simulink model "new"  (R2025a)
settings: Solver=VariableStepAuto  StartTime=0.0  StopTime=10.0  RelTol=1e-3
settings Model: Creator=nasim  LastModifiedBy=nasim

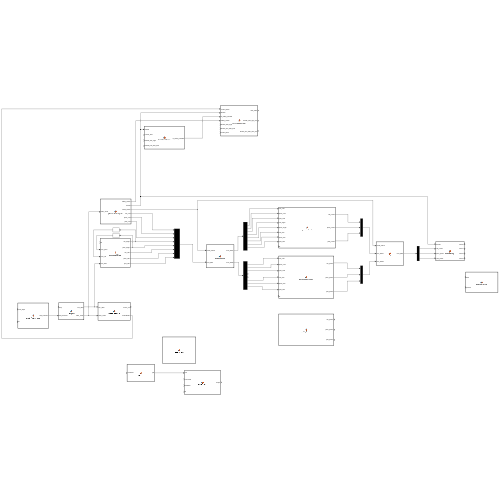
[thumbnail: Simulink's stored preview of the top-level diagram]
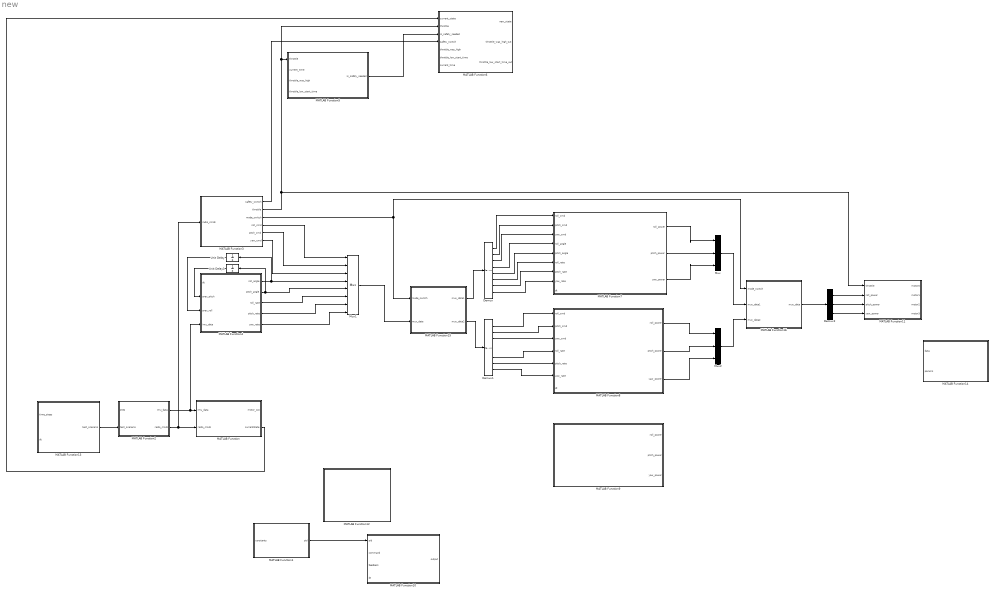
== system new ==
  Demux : Demux  Outputs=8
  Demux1 : Demux  Outputs=8
  Demux2 : Demux  Outputs=3
  MATLAB Function : MATLAB Function  TreatAsAtomicUnit=on
  MATLAB Function1 : MATLAB Function  TreatAsAtomicUnit=on
  MATLAB Function10 : MATLAB Function  TreatAsAtomicUnit=on
  MATLAB Function11 : MATLAB Function  TreatAsAtomicUnit=on
  MATLAB Function12 : MATLAB Function  TreatAsAtomicUnit=on
  MATLAB Function13 : MATLAB Function  TreatAsAtomicUnit=on
  MATLAB Function14 : MATLAB Function  TreatAsAtomicUnit=on
  MATLAB Function15 : MATLAB Function  TreatAsAtomicUnit=on
  MATLAB Function16 : MATLAB Function  TreatAsAtomicUnit=on
  MATLAB Function2 : MATLAB Function  TreatAsAtomicUnit=on
  MATLAB Function3 : MATLAB Function  TreatAsAtomicUnit=on
  MATLAB Function4 : MATLAB Function  TreatAsAtomicUnit=on
  MATLAB Function5 : MATLAB Function  TreatAsAtomicUnit=on
  MATLAB Function6 : MATLAB Function  TreatAsAtomicUnit=on
  MATLAB Function7 : MATLAB Function  TreatAsAtomicUnit=on
  MATLAB Function8 : MATLAB Function  TreatAsAtomicUnit=on
  MATLAB Function9 : MATLAB Function  TreatAsAtomicUnit=on
  Mux : Mux  Inputs=3
  Mux1 : Mux  Inputs=8
  Mux2 : Mux  Inputs=3
  Unit Delay : UnitDelay  SampleTime=-1  HasFrameUpgradeWarning=on
  Unit Delay1 : UnitDelay  SampleTime=-1  HasFrameUpgradeWarning=on
  wires:
  MATLAB Function2/1(imu_data) -> MATLAB Function/1(imu_data), MATLAB Function4/4(imu_data)
  MATLAB Function2/2(radio_cmds) -> MATLAB Function/2(radio_cmds), MATLAB Function3/1(radio_cmds)
  MATLAB Function3/2(throttle) -> MATLAB Function6/2(throttle), MATLAB Function5/1(throttle), MATLAB Function11/1(throttle)
  MATLAB Function/2(currentState) -> MATLAB Function6/1(current_state)
  MATLAB Function5/1(is_safety_needed) -> MATLAB Function6/3(is_safety_needed)
  MATLAB Function3/1(safety_switch) -> MATLAB Function6/4(safety_switch)
  MATLAB Function13/1(test_scenario) -> MATLAB Function2/2(test_scenario)
  MATLAB Function1/1(pid) -> MATLAB Function10/1(pid)
  Mux1/1 -> MATLAB Function15/2(mux_data)
  MATLAB Function3/3(mode_switch) -> MATLAB Function16/1(mode_switch), MATLAB Function15/1(mode_switch)
  MATLAB Function15/1(mux_data1) -> Demux/1
  MATLAB Function15/2(mux_data2) -> Demux1/1
  MATLAB Function7/1(roll_power) -> Mux/1
  MATLAB Function7/2(pitch_power) -> Mux/2
  MATLAB Function7/3(yaw_power) -> Mux/3
  MATLAB Function8/1(roll_power) -> Mux2/1
  MATLAB Function8/2(pitch_power) -> Mux2/2
  MATLAB Function8/3(yaw_power) -> Mux2/3
  MATLAB Function16/1(mux_data) -> Demux2/1
  Demux2/1 -> MATLAB Function11/2(roll_power)
  Demux2/2 -> MATLAB Function11/3(pitch_power)
  Demux2/3 -> MATLAB Function11/4(yaw_power)
  Mux/1 -> MATLAB Function16/2(mux_data1)
  Mux2/1 -> MATLAB Function16/3(mux_data2)
  MATLAB Function3/4(roll_cmd) -> Mux1/1
  MATLAB Function3/5(pitch_cmd) -> Mux1/2
  MATLAB Function3/6(yaw_cmd) -> Mux1/3
  MATLAB Function4/1(roll_angle) -> Mux1/4, Unit Delay/1
  MATLAB Function4/2(pitch_angle) -> Mux1/5, Unit Delay1/1
  MATLAB Function4/3(roll_rate) -> Mux1/6
  MATLAB Function4/4(pitch_rate) -> Mux1/7
  MATLAB Function4/5(yaw_rate) -> Mux1/8
  Demux/2 -> MATLAB Function7/2(pitch_cmd)
  Demux/3 -> MATLAB Function7/3(yaw_cmd)
  Demux/4 -> MATLAB Function7/4(roll_angle)
  Demux/1 -> MATLAB Function7/1(roll_cmd)
  Demux/5 -> MATLAB Function7/5(pitch_angle)
  Demux/6 -> MATLAB Function7/6(roll_rate)
  Demux/7 -> MATLAB Function7/7(pitch_rate)
  Demux/8 -> MATLAB Function7/8(yaw_rate)
  Demux1/1 -> MATLAB Function8/1(roll_cmd)
  Demux1/2 -> MATLAB Function8/2(pitch_cmd)
  Demux1/3 -> MATLAB Function8/3(yaw_cmd)
  Demux1/6 -> MATLAB Function8/4(roll_rate)
  Demux1/7 -> MATLAB Function8/5(pitch_rate)
  Demux1/8 -> MATLAB Function8/6(yaw_rate)
  Unit Delay/1 -> MATLAB Function4/3(prev_roll)
  Unit Delay1/1 -> MATLAB Function4/2(prev_pitch)

== matlab function new/MATLAB Function8 ==
  data: roll_cmd input; pitch_cmd input; yaw_cmd input; roll_rate input; pitch_rate input; yaw_rate input; roll_power output; dt input; pitch_power output; yaw_power output
function [roll_power, pitch_power, yaw_power] = accroModeControl(roll_cmd, pitch_cmd, yaw_cmd,roll_rate, pitch_rate, yaw_rate, dt)
    % Accro mode control - single PID (from Stabilization::Accro)
    persistent rollSpeedPID_Accro pitchSpeedPID_Accro yawPID;
    global params;
    
    if isempty(rollSpeedPID_Accro)
        rollSpeedPID_Accro = initPID(params.accroSpeed);
        pitchSpeedPID_Accro = initPID(params.accroSpeed);
        yawPID = initPID(params.yawSpeed);
    end
    
    % Direct rate control
    roll_power = computePID(rollSpeedPID_Accro, roll_cmd, roll_rate, dt);
    pitch_power = computePID(pitchSpeedPID_Accro, pitch_cmd, pitch_rate, dt);
    yaw_power = computePID(yawPID, yaw_cmd, yaw_rate, dt);
end

== matlab function new/MATLAB Function9 ==
  data: roll_power output; pitch_power output; yaw_power output
function [roll_power, pitch_power, yaw_power] = safetyControl()
    % Safety control - all motors idle (from Stabilization::Idle)
    roll_power = 0;
    pitch_power = 0;
    yaw_power = 0;
    
    % Reset all PID controllers
    resetAllPIDs();
end

== matlab function new/MATLAB Function10 ==
  data: pid input; output output; command input; feedback input; dt input
function output = computePID(pid, command, feedback, dt)
    % Generic PID computation (from ControlLoop::ComputeCorrection)
    error = command - feedback;
    pid.integrator = pid.integrator + error;
    
    output = pid.G * (pid.Kp * error + pid.Kd * (error - pid.prev_error) / dt + pid.Ki * pid.integrator);
    
    pid.prev_error = error;
end

== matlab function new/MATLAB Function11 ==
  data: throttle input; roll_power input; pitch_power input; yaw_power input; motor0 output; motor1 output; motor2 output; motor3 output
function [motor0, motor1, motor2, motor3] = motorMixing(throttle, roll_power, pitch_power, yaw_power)
    % X-configuration motor mixing (from Stabilization::SetMotorsPwrXConfig)
    global params;
    
    % Convert throttle percentage to PWM
    throttle_pwm = params.MOTOR_MIN_POWER + (throttle / 100) * (params.MOTOR_MAX_POWER - params.MOTOR_MIN_POWER);
    
    % X configuration mixing
    motor0 = throttle_pwm - pitch_power * params.mixing + roll_power * params.mixing - yaw_power * params.mixing;
    motor1 = throttle_pwm - pitch_power * params.mixing - roll_power * params.mixing + yaw_power * params.mixing;
    motor2 = throttle_pwm + pitch_power * params.mixing - roll_power * params.mixing - yaw_power * params.mixing;
    motor3 = throttle_pwm + pitch_power * params.mixing + roll_power * params.mixing + yaw_power * params.mixing;
    
    % Apply PWM limits
    motor0 = max(params.MOTOR_MIN_POWER, min(params.MOTOR_MAX_POWER, motor0));
    motor1 = max(params.MOTOR_MIN_POWER, min(params.MOTOR_MAX_POWER, motor1));
    motor2 = max(params.MOTOR_MIN_POWER, min(params.MOTOR_MAX_POWER, motor2));
    motor3 = max(params.MOTOR_MIN_POWER, min(params.MOTOR_MAX_POWER, motor3));
end

== matlab function new/MATLAB Function12 ==
function resetAllPIDs()
    % Reset all PID controllers (from Stabilization::ResetPID)
    persistent rollPosPID pitchPosPID rollSpeedPID_Angle pitchSpeedPID_Angle;
    persistent rollSpeedPID_Accro pitchSpeedPID_Accro yawPID;
    
    if ~isempty(rollPosPID)
        rollPosPID.integrator = 0;
        rollPosPID.prev_error = 0;
    end
    if ~isempty(pitchPosPID)
        pitchPosPID.integrator = 0;
        pitchPosPID.prev_error = 0;
    end
    if ~isempty(rollSpeedPID_Angle)
        rollSpeedPID_Angle.integrator = 0;
        rollSpeedPID_Angle.prev_error = 0;
    end
    if ~isempty(pitchSpeedPID_Angle)
        pitchSpeedPID_Angle.integrator = 0;
        pitchSpeedPID_Angle.prev_error = 0;
    end
    if ~isempty(rollSpeedPID_Accro)
        rollSpeedPID_Accro.integrator = 0;
        rollSpeedPID_Accro.prev_error = 0;
    end
    if ~isempty(pitchSpeedPID_Accro)
        pitchSpeedPID_Accro.integrator = 0;
        pitchSpeedPID_Accro.prev_error = 0;
    end
    if ~isempty(yawPID)
        yawPID.integrator = 0;
        yawPID.prev_error = 0;
    end
end

== matlab function new/MATLAB Function13 ==
  data: time_steps input; test_scenario output; dt input
function test_scenario = createTestScenario(time_steps, dt)
    % Create test scenario with realistic inputs
    time = (0:time_steps-1) * dt;
    
    % Radio commands
    test_scenario.roll_raw = 1500 + 200 * sin(2*pi*0.1*time);     % Slow roll oscillation
    test_scenario.pitch_raw = 1500 + 150 * sin(2*pi*0.15*time);   % Pitch oscillation
    test_scenario.throttle_raw = 1090 + 0 * (time < 5) + 200 * (time >= 5 & time < 15) + 400 * (time >= 15); % Step throttle: 1090->1090->1290->1490
    test_scenario.yaw_raw = 1500 + 100 * sin(2*pi*0.05*time);     % Slow yaw
    test_scenario.mode_raw = 1900 * ones(size(time));             % Angle mode
    test_scenario.safety_raw = 1900 * ones(size(time));           % Armed
    
    % IMU data (simulated)
    test_scenario.acc_x = 0.1 * sin(2*pi*0.1*time);              % Small accelerations
    test_scenario.acc_y = 0.15 * sin(2*pi*0.15*time);
    test_scenario.acc_z = 9.81 + 0.05 * sin(2*pi*0.05*time);     % Gravity + noise
    
    test_scenario.gyro_x = 2 * sin(2*pi*0.1*time);               % Gyro rates
    test_scenario.gyro_y = 1.5 * sin(2*pi*0.15*time);
    test_scenario.gyro_z = 0.5 * sin(2*pi*0.05*time);
end

== matlab function new/MATLAB Function14 ==
  data: data input; params input
function analyzeResults(data, params)
    % Analyze and plot simulation results
    figure('Name', 'CodeDroneDIY Simulation Results', 'Position', [100, 100, 1200, 800]);
    
    % Time vector
    time = data.time;
    
    % Plot 1: Attitude
    subplot(3, 3, 1);
    plot(time, data.roll_angle, 'r-', time, data.pitch_angle, 'b-', 'LineWidth', 2);
    xlabel('Time (s)'); ylabel('Angle (deg)');
    title('Attitude Angles'); legend('Roll', 'Pitch'); grid on;
    
    % Plot 2: Angular Rates
    subplot(3, 3, 2);
    plot(time, data.roll_rate, 'r-', time, data.pitch_rate, 'b-', time, data.yaw_rate, 'g-', 'LineWidth', 2);
    xlabel('Time (s)'); ylabel('Rate (deg/s)');
    title('Angular Rates'); legend('Roll', 'Pitch', 'Yaw'); grid on;
    
    % Plot 3: Commands
    subplot(3, 3, 3);
    plot(time, data.roll_cmd, 'r-', time, data.pitch_cmd, 'b-', 'LineWidth', 2);
    xlabel('Time (s)'); ylabel('Command (deg)');
    title('Control Commands'); legend('Roll Cmd', 'Pitch Cmd'); grid on;
    
    % Plot 4: Throttle
    subplot(3, 3, 4);
    plot(time, data.throttle, 'k-', 'LineWidth', 2);
    xlabel('Time (s)'); ylabel('Throttle (%)');
    title('Throttle'); grid on;
    
    % Plot 5: Motor Outputs
    subplot(3, 3, 5);
    plot(time, data.motor0, 'r-', time, data.motor1, 'g-', time, data.motor2, 'b-', time, data.motor3, 'k-', 'LineWidth', 2);
    xlabel('Time (s)'); ylabel('PWM (us)');
    title('Motor Outputs'); legend('Motor0', 'Motor1', 'Motor2', 'Motor3'); grid on;
    
    % Plot 6: State Machine
    subplot(3, 3, 6);
    plot(time, data.state, 'k-', 'LineWidth', 2);
    xlabel('Time (s)'); ylabel('State');
    title('State Machine'); ylim([0, 6]); grid on;
    
    % Plot 7: Loop Timing
    subplot(3, 3, 7);
    plot(time, data.loop_time * 1000, 'b-', 'LineWidth', 2);
    hold on;
    plot(time, params.LOOP_TIME_TARGET * 1000 * ones(size(time)), 'r--', 'LineWidth', 2);
    xlabel('Time (s)'); ylabel('Loop Time (ms)');
    title('Loop Timing'); legend('Actual', 'Target'); grid on;
    
    % Plot 8: Control Performance
    subplot(3, 3, 8);
    plot(time, data.roll_cmd - data.roll_angle, 'r-', time, data.pitch_cmd - data.pitch_angle, 'b-', 'LineWidth', 2);
    xlabel('Time (s)'); ylabel('Error (deg)');
    title('Control Errors'); legend('Roll Error', 'Pitch Error'); grid on;
    
    % Plot 9: Power Analysis
    subplot(3, 3, 9);
    total_power = data.motor0 + data.motor1 + data.motor2 + data.motor3;
    plot(time, total_power, 'k-', 'LineWidth', 2);
    xlabel('Time (s)'); ylabel('Total Power (us)');
    title('Total Motor Power'); grid on;
    
    % Print performance summary
    fprintf('\n=== PERFORMANCE ANALYSIS ===\n');
    fprintf('RMS Roll Error: %.2f degrees\n', rms(data.roll_cmd - data.roll_angle));
    fprintf('RMS Pitch Error: %.2f degrees\n', rms(data.pitch_cmd - data.pitch_angle));
    fprintf('Mean Loop Time: %.3f ms (Target: %.3f ms)\n', mean(data.loop_time)*1000, params.LOOP_TIME_TARGET*1000);
    fprintf('Loop Time Std: %.3f ms\n', std(data.loop_time)*1000);
    fprintf('Max Loop Time: %.3f ms\n', max(data.loop_time)*1000);
end

== matlab function new/MATLAB Function1 ==
  data: constants input; pid output
function pid = initPID(constants)
    % Initialize PID controller structure
    pid = struct();
    pid.G = constants.G;
    pid.Kp = constants.Kp;
    pid.Kd = constants.Kd;
    pid.Ki = constants.Ki;
    pid.integrator = 0;
    pid.prev_error = 0;
end

== matlab function new/MATLAB Function15 ==
  data: mode_switch input; mux_data1 output; mux_data input; mux_data2 output
function [mux_data1, mux_data2] = modeSelector(mode_switch, mux_data)
% This function routes the input bus 'mux_data' to one of two outputs
% based on the 'mode_switch' signal.

% Ensure the output ports are the same size and type as the input port.
% This is crucial for Simulink to understand the data types.
% coder.varsize('mux_data1', 'mux_data2'); % Optional, but good practice

if mode_switch ~= 0
    % If mode_switch is active (e.g., 1 for Angle Mode),
    % route data to the first output.
    mux_data1 = mux_data;
    
    % The second output receives a zero or empty signal of the same type.
    mux_data2 = 0 * mux_data; % Creates a zero-filled bus of the same structure
else
    % If mode_switch is inactive (0 for Accro Mode),
    % the first output gets the zero signal.
    mux_data1 = 0 * mux_data; 
    
    % Route the data to the second output.
    mux_data2 = mux_data;
end

== matlab function new/MATLAB Function16 ==
  data: mode_switch input; mux_data output; mux_data1 input; mux_data2 input
function mux_data  = modefnc(mode_switch, mux_data1, mux_data2)
if mode_switch ~= 0
    mux_data = mux_data1;
    
else
    mux_data = mux_data2; 
    
end

== matlab function new/MATLAB Function ==
  data: imu_data input; radio_cmds input; motor_out output; currentState output
function [motor_out, currentState] = DroneController(imu_data, radio_cmds)
% This function implements the drone flight controller logic for a single time step.

%#codegen

% Declare persistent variables to hold state between function calls
persistent rollPosPID pitchPosPID rollSpeedPID_Angle pitchSpeedPID_Angle;
persistent rollSpeedPID_Accro pitchSpeedPID_Accro yawPID;
persistent roll_angle_filt pitch_angle_filt;
persistent throttle_was_high throttle_low_start_time;
persistent currentState_internal;

% Load parameters from the base workspace
coder.extrinsic('evalin'); % Allow access to base workspace
params = evalin('base', 'params');

% Initialize all persistent variables on the first run
if isempty(currentState_internal)
    % Initialize PID controllers
    rollPosPID          = initPID(params.anglePos);
    pitchPosPID         = initPID(params.anglePos);
    rollSpeedPID_Angle  = initPID(params.angleSpeed);
    pitchSpeedPID_Angle = initPID(params.angleSpeed);
    rollSpeedPID_Accro  = initPID(params.accroSpeed);
    pitchSpeedPID_Accro = initPID(params.accroSpeed);
    yawPID              = initPID(params.yawSpeed);
    
    % Initialize attitude filter states
    roll_angle_filt     = 0;
    pitch_angle_filt    = 0;
    
    % Initialize safety logic states
    throttle_was_high       = true;
    throttle_low_start_time = 0;
    
    % Initialize state machine
    currentState_internal = params.states.INITIALIZING;
end

% Get simulation time and time step (dt)
current_time = get_param(bdroot, 'SimulationTime');
dt = params.LOOP_TIME_TARGET; % Assumes fixed-step solver

% -------------------- LOGIC FROM YOUR FOR LOOP --------------------

% 1. Process radio inputs
[roll_cmd, pitch_cmd, throttle, yaw_cmd, ~, safety_switch] = processRadioInputs(radio_cmds, params);

% 2. Process IMU data
[roll_angle, pitch_angle, roll_rate, pitch_rate, yaw_rate] = processIMUData(imu_data, dt, roll_angle_filt, pitch_angle_filt, params);

% Update filtered angles for the next time step
roll_angle_filt = roll_angle;
pitch_angle_filt = pitch_angle;

% 3. Check safety conditions
is_safety_needed = checkSafetyState(throttle, current_time, throttle_was_high, throttle_low_start_time);

% 4. Run State Machine
[new_state, throttle_was_high, throttle_low_start_time] = runStateMachine(currentState_internal, throttle, is_safety_needed, safety_switch, throttle_was_high, throttle_low_start_time, current_time, params);
currentState_internal = new_state;

% 5. Run Control Logic based on state
roll_motor_power = 0;
pitch_motor_power = 0;
yaw_motor_power = 0;

switch currentState_internal
    case params.states.ANGLEMODE
        % Angle mode - cascaded PID
        [roll_motor_power, pitch_motor_power, yaw_motor_power] = angleModeControl(...
            roll_cmd, pitch_cmd, yaw_cmd, ...
            roll_angle, pitch_angle, roll_rate, pitch_rate, yaw_rate, dt, ...
            rollPosPID, pitchPosPID, rollSpeedPID_Angle, pitchSpeedPID_Angle, yawPID);
        
    case params.states.ACCRONODE
        % Accro mode - speed PID
        [roll_motor_power, pitch_motor_power, yaw_motor_power] = accroModeControl(...
            roll_cmd, pitch_cmd, yaw_cmd, ...
            roll_rate, pitch_rate, yaw_rate, dt, ...
            rollSpeedPID_Accro, pitchSpeedPID_Accro, yawPID);
        
    case {params.states.SAFETY, params.states.DISARMED, params.states.INITIALIZING}
        % Safety states - reset controllers and output zero power
        [roll_motor_power, pitch_motor_power, yaw_motor_power] = safetyControl();
        % Also reset PID integrators
        rollPosPID.integral = 0; pitchPosPID.integral = 0;
        rollSpeedPID_Angle.integral = 0; pitchSpeedPID_Angle.integral = 0;
        rollSpeedPID_Accro.integral = 0; pitchSpeedPID_Accro.integral = 0;
        yawPID.integral = 0;
end

% 6. X-configuration motor mixing
[m0, m1, m2, m3] = motorMixing(throttle, roll_motor_power, pitch_motor_power, yaw_motor_power, params);

% 7. Assign outputs for the Simulink block
motor_out = [m0; m1; m2; m3];
currentState = currentState_internal;

end


% -------------------- HELPER FUNCTIONS --------------------
% All your other functions (initPID, processRadioInputs, etc.) go here
% as local functions. Make sure they are self-contained.

function pid = initPID(p)
    pid = struct('G', p.G, 'Kp', p.Kp, 'Kd', p.Kd, 'Ki', p.Ki, ...
                 'integral', 0, 'previous_error', 0);
end

function [roll_cmd, pitch_cmd, throttle, yaw_cmd, mode_switch, safety_switch] = processRadioInputs(radio_cmds, params)
    % Dummy function - replace with your actual mapping logic
    throttle = radio_cmds(1); % Assuming throttle is the first channel
    roll_cmd = map_input(radio_cmds(2), params.MAX_ANGLE);
    pitch_cmd = map_input(radio_cmds(3), params.MAX_ANGLE);
    yaw_cmd = map_input(radio_cmds(4), params.MAX_YAW_SPEED);
    mode_switch = radio_cmds(5);
    safety_switch = radio_cmds(6);
end

function out = map_input(value, max_value)
    % Maps a generic input (e.g., 1000-2000) to a physical value
    out = (value - 1500) / 500 * max_value;
end

% ... include all your other helper functions here ...
% e.g., processIMUData, checkSafetyState, runStateMachine, angleModeControl, 
% accroModeControl, safetyControl, motorMixing, etc.

== matlab function new/MATLAB Function2 ==
  data: imu_data output; step input; test_scenario input; radio_cmds output
function [imu_data, radio_cmds] = getInputs(step, test_scenario)
    % Get inputs from test scenario (replace with real sensor data)
    radio_cmds = struct();
    radio_cmds.roll = test_scenario.roll_raw(step);
    radio_cmds.pitch = test_scenario.pitch_raw(step);
    radio_cmds.throttle = test_scenario.throttle_raw(step);
    radio_cmds.yaw = test_scenario.yaw_raw(step);
    radio_cmds.mode = test_scenario.mode_raw(step);
    radio_cmds.safety = test_scenario.safety_raw(step);
    
    imu_data = struct();
    imu_data.acc_x = test_scenario.acc_x(step);
    imu_data.acc_y = test_scenario.acc_y(step);
    imu_data.acc_z = test_scenario.acc_z(step);
    imu_data.gyro_x = test_scenario.gyro_x(step);
    imu_data.gyro_y = test_scenario.gyro_y(step);
    imu_data.gyro_z = test_scenario.gyro_z(step);
end

== matlab function new/MATLAB Function3 ==
  data: safety_switch output; throttle output; mode_switch output; radio_cmds input; roll_cmd output; pitch_cmd output; yaw_cmd output
function [safety_switch, throttle,mode_switch,  roll_cmd, pitch_cmd, yaw_cmd] = processRadioInputs(radio_cmds)
    % Process radio inputs (from RadioReception.cpp)
    global params;
    
    % Scale inputs to match your C++ code
    roll_cmd = (radio_cmds.roll - 1500) * params.MAX_ANGLE / 400;      % ±45 degrees
    pitch_cmd = (radio_cmds.pitch - 1500) * params.MAX_ANGLE / 400;    % ±45 degrees
    throttle = (radio_cmds.throttle - 1090) * 100 / 810; % 0-100%
    yaw_cmd = (radio_cmds.yaw - 1500) * params.MAX_YAW_SPEED / 400;       % ±135 deg/s
    
    % Mode selection
    if radio_cmds.mode > 1700
        mode_switch = 1; % Angle mode
    elseif radio_cmds.mode < 1300
        mode_switch = 0; % Accro mode
    else
        mode_switch = 0; % Default to Accro
    end
    
    % Safety switch
    safety_switch = (radio_cmds.safety > 1500);
    
    % Apply limits
    roll_cmd = max(-params.MAX_ANGLE, min(params.MAX_ANGLE, roll_cmd));
    pitch_cmd = max(-params.MAX_ANGLE, min(params.MAX_ANGLE, pitch_cmd));
    yaw_cmd = max(-params.MAX_YAW_SPEED, min(params.MAX_YAW_SPEED, yaw_cmd));
    throttle = max(0, min(100, throttle));
end

== matlab function new/MATLAB Function4 ==
  data: dt input; prev_pitch input; prev_roll input; imu_data input; roll_angle output; pitch_angle output; roll_rate output; pitch_rate output; yaw_rate output
function [roll_angle, pitch_angle, roll_rate, pitch_rate, yaw_rate] = processIMUData(dt, prev_pitch, prev_roll, imu_data)
    % Process IMU data with complementary filter (from Stabilization.cpp)
    global params;
    
    % Convert gyro to degrees/second
    roll_rate = imu_data.gyro_x;
    pitch_rate = imu_data.gyro_y;
    yaw_rate = imu_data.gyro_z;
    
    % Normalize accelerometer
    acc_mag = sqrt(imu_data.acc_x^2 + imu_data.acc_y^2 + imu_data.acc_z^2);
    acc_x_norm = imu_data.acc_x / acc_mag;
    acc_y_norm = imu_data.acc_y / acc_mag;
    acc_z_norm = imu_data.acc_z / acc_mag;
    
    % Calculate angles from accelerometer
    roll_angle_acc = atan2(acc_y_norm, acc_z_norm) * 180/pi;
    pitch_angle_acc = atan2(-acc_x_norm, acc_z_norm) * 180/pi;
    
    % Complementary filter (from Stabilization::ApplyComplementaryFilter)
    roll_angle = params.HighPassFilterCoeff * (prev_roll + roll_rate * dt) + (1 - params.HighPassFilterCoeff) * roll_angle_acc;
    pitch_angle = params.HighPassFilterCoeff * (prev_pitch + pitch_rate * dt) + (1 - params.HighPassFilterCoeff) * pitch_angle_acc;
end

== matlab function new/MATLAB Function5 ==
  data: throttle input; is_safety_needed output; current_time input; throttle_was_high input; throttle_low_start_time input
function is_safety_needed = checkSafetyState(throttle, current_time, throttle_was_high, throttle_low_start_time)
    % Safety state logic (from StateMachine::IsSafetyStateNeeded)
    global params;
    
    if throttle_was_high && throttle < params.MOTOR_IDLE_THRESHOLD
        is_safety_needed = false;
    elseif ~throttle_was_high && (current_time - throttle_low_start_time > params.SAFETY_TIMEOUT)
        is_safety_needed = true;
    else
        is_safety_needed = false;
    end
end

== matlab function new/MATLAB Function6 ==
  data: current_state input; new_state output; throttle input; is_safety_needed input; safety_switch input; throttle_was_high input; throttle_low_start_time input; current_time input; throttle_was_high_out output; throttle_low_start_time_out output
function [new_state, throttle_was_high_out, throttle_low_start_time_out] = runStateMachine(current_state, throttle, is_safety_needed, safety_switch, throttle_was_high, throttle_low_start_time, current_time)
    % State machine logic (from StateMachine.cpp and state implementations)
    global params;
    
    new_state = current_state;
    throttle_was_high_out = throttle_was_high;
    throttle_low_start_time_out = throttle_low_start_time;
    
    switch current_state
        case params.states.INITIALIZING
            % Transition to Disarmed when IMU is calibrated (from Initializing.cpp)
            % In the C++ code, this transitions to Disarmed, then to AngleMode when throttle high
            new_state = params.states.DISARMED;
            
        case params.states.ANGLEMODE
            if is_safety_needed
                new_state = params.states.SAFETY;
            end
            
        case params.states.ACCRONODE
            if is_safety_needed
                new_state = params.states.SAFETY;
            end
            
        case params.states.SAFETY
            % Automatic transition to disarmed after 1 second
            new_state = params.states.DISARMED;
            
        case params.states.DISARMED
            % Transition back to armed when throttle high and safety switch on
            if throttle > params.MOTOR_IDLE_THRESHOLD && safety_switch
                new_state = params.states.ANGLEMODE;
            end
    end
    
    % Update throttle tracking
    if throttle_was_high && throttle < params.MOTOR_IDLE_THRESHOLD
        throttle_was_high_out = false;
        throttle_low_start_time_out = current_time;
    elseif throttle > params.MOTOR_IDLE_THRESHOLD
        throttle_was_high_out = true;
    end
end

== matlab function new/MATLAB Function7 ==
  data: roll_cmd input; pitch_cmd input; yaw_cmd input; roll_angle input; pitch_angle input; roll_rate input; pitch_rate input; yaw_rate input; roll_power output; dt input; pitch_power output; yaw_power output
function [roll_power, pitch_power, yaw_power] = angleModeControl(roll_cmd, pitch_cmd, yaw_cmd, roll_angle, pitch_angle, roll_rate, pitch_rate, yaw_rate,  dt)
    % Angle mode control - cascaded PID (from Stabilization::Angle)
    persistent rollPosPID pitchPosPID rollSpeedPID_Angle pitchSpeedPID_Angle yawPID;
    global params;
    
    if isempty(rollPosPID)
        rollPosPID = initPID(params.anglePos);
        pitchPosPID = initPID(params.anglePos);
        rollSpeedPID_Angle = initPID(params.angleSpeed);
        pitchSpeedPID_Angle = initPID(params.angleSpeed);
        yawPID = initPID(params.yawSpeed);
    end
    
    % Roll control - cascaded PID
    roll_pos_cmd = computePID(rollPosPID, roll_cmd, roll_angle, dt);
    roll_power = computePID(rollSpeedPID_Angle, roll_pos_cmd, roll_rate, dt);
    
    % Pitch control - cascaded PID
    pitch_pos_cmd = computePID(pitchPosPID, pitch_cmd, pitch_angle, dt);
    pitch_power = computePID(pitchSpeedPID_Angle, pitch_pos_cmd, pitch_rate, dt);
    
    % Yaw control - single PID (always rate control)
    yaw_power = computePID(yawPID, yaw_cmd, yaw_rate, dt);
end
